simulink model "Project1_part2_opt1_spring"  (R2025b)
settings: Solver=ode45  StartTime=0.0  StopTime=25  FixedStep=1  RelTol=1e-3
values from neighbouring files (symbols this model uses):
  b1 = 1    [run_project1_part2_op3.m]    (also in run_project1_part2_opt1.m; run_project1_part2_opt2.m)
  b2 = 1    [run_project1_part2_op3.m]    (also in run_project1_part2_opt1.m; run_project1_part2_opt2.m)
  J1 = 100    [run_project1_part2_op3.m]    (also in run_project1_part2_opt1.m; run_project1_part2_opt2.m)
  J2 = 1    [run_project1_part2_op3.m]    (also in run_project1_part2_opt1.m; run_project1_part2_opt2.m)
  omega10 = 0    [run_project1_part2_opt1.m]
  omega20 = 0    [run_project1_part2_opt1.m]
  theta10 = 0    [run_project1_part2_opt1.m]
  theta20 = 0    [run_project1_part2_opt1.m]
undefined symbols (not defined in the file or in its folder): A, k
settings Model: Creator=KI5UXW  LastModifiedBy=KI5UXW

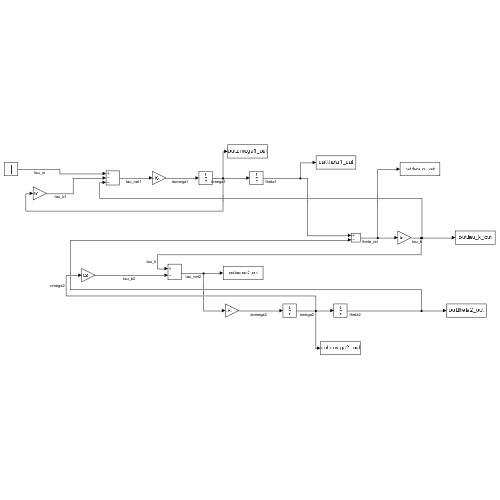
[thumbnail: Simulink's stored preview of the top-level diagram]
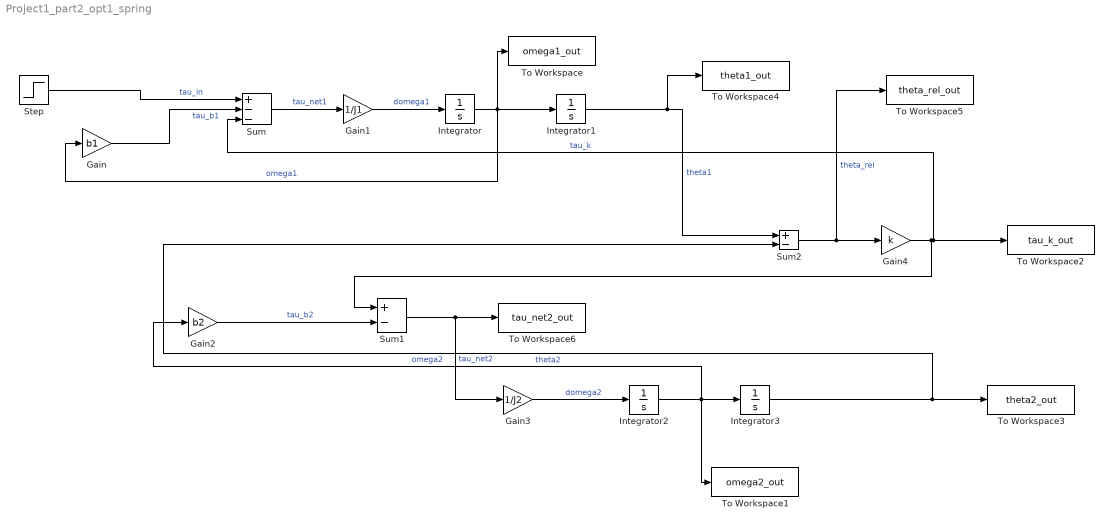
== system Project1_part2_opt1_spring ==
  Gain : Gain  Gain=b1
  Gain1 : Gain  Gain=1/J1
  Gain2 : Gain  Gain=b2
  Gain3 : Gain  Gain=1/J2
  Gain4 : Gain  Gain=k
  Integrator : Integrator  InitialCondition=omega10
  Integrator1 : Integrator  InitialCondition=theta10
  Integrator2 : Integrator  InitialCondition=omega20
  Integrator3 : Integrator  InitialCondition=theta20
  Step : Step  Time=0  After=A  SampleTime=0
  Sum : Sum  Inputs=+--
  Sum1 : Sum  Inputs=+-
  Sum2 : Sum  Inputs=+-
  To Workspace : ToWorkspace  VariableName=omega1_out  SaveFormat=Timeseries  SampleTime=-1
  To Workspace1 : ToWorkspace  VariableName=omega2_out  SaveFormat=Timeseries  SampleTime=-1
  To Workspace2 : ToWorkspace  VariableName=tau_k_out  SaveFormat=Timeseries  SampleTime=-1
  To Workspace3 : ToWorkspace  VariableName=theta2_out  SaveFormat=Timeseries  SampleTime=-1
  To Workspace4 : ToWorkspace  VariableName=theta1_out  SaveFormat=Timeseries  SampleTime=-1
  To Workspace5 : ToWorkspace  VariableName=theta_rel_out  SaveFormat=Timeseries  SampleTime=-1
  To Workspace6 : ToWorkspace  VariableName=tau_net2_out  SaveFormat=Timeseries  SampleTime=-1
  wires:
  Step/1 -> Sum/1  "tau_in"
  Gain/1 -> Sum/2  "tau_b1"
  Sum/1 -> Gain1/1  "tau_net1"
  Gain1/1 -> Integrator/1  "domega1"
  Integrator/1 -> To Workspace/1, Gain/1, Integrator1/1  "omega1"
  Integrator1/1 -> To Workspace4/1, Sum2/1  "theta1"
  Gain2/1 -> Sum1/2  "tau_b2"
  Gain4/1 -> Sum/3, To Workspace2/1, Sum1/1  "tau_k"
  Gain3/1 -> Integrator2/1  "domega2"
  Integrator2/1 -> To Workspace1/1, Gain2/1, Integrator3/1  "omega2"
  Integrator3/1 -> Sum2/2, To Workspace3/1  "theta2"
  Sum2/1 -> To Workspace5/1, Gain4/1  "theta_rel"
  Sum1/1 -> To Workspace6/1, Gain3/1  "tau_net2"
